simulink model "ship"  (Simulink 9.2)
settings: Solver=ode45  StartTime=0.0  StopTime=500  RelTol=1e-3  EnableMultiTasking=on
values from neighbouring files (symbols this model uses):
  K_pd = 0.8362    [variables.mat]
  psi_r = 30    [variables.mat]
  T_d = 72.5216    [variables.mat]
  T_f = 8.39    [variables.mat]
libraries: simulink x2, simulink_extras x2
settings Model: Creator=markh  LastModifiedBy=Kjetk
settings DataIOCC: SignalLoggingName=sigsOut
settings OptimizationCC: InitFltsAndDblsToZero=on
settings DebuggingCC: SaveWithParameterizedLinksMsg=none  SignalResolutionControl=TryResolveAllWithWarning  MultiTaskDSMMsg=warning  MultiTaskCondExecSysMsg=none
settings HardwareCC: TargetUnknown=on
settings GRTTargetCC: TargetFcnLib=ansi_tfl_tmw.mat

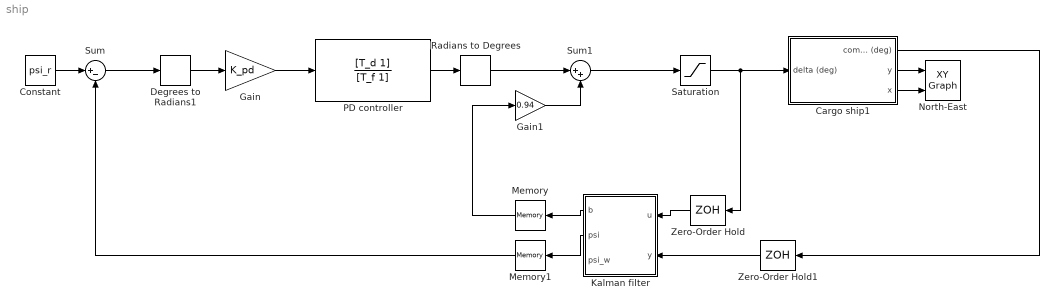
== system ship ==
  Cargo ship1 : Subsystem  mask(Simple shipmodel for a cargo ship){noise=on, current=on, logic=off}
      mask prompts: noise "measurement noise"; logic "waves"
      mask help:
      | Measurement noise:
      | 	checked = noise on
      | 	unchecked = noise off
      |
      | Current:
      | 	checked = current on
      | 	unchecked = current off
      |
      | Waves:
      | 	checked = waves on
      | 	unchecked = waves off
      |
      | Author: Jørgen Spjøtvold, 9/10-2003
      | TTK 4115 Linear system theory.
      | Modified by Jostein Bakkeheim 26/10-2006
  Constant : Constant  Value=psi_r
  Degrees to Radians1 : simulink_extras/Transformations/Degrees to Radians
  Gain : Gain  Gain=K_pd
  Gain1 : Gain  Gain=0.94
  Kalman filter : MATLAB Function  TreatAsAtomicUnit=on
  Memory : Memory
  Memory1 : Memory
  "North-East " : simulink/Sinks/XY Graph  xmin=-1  xmax=1  ymin=-1  ymax=1  st=-1
  PD controller : TransferFcn  Numerator=[T_d 1]  Denominator=[T_f 1]
  Radians to Degrees : simulink_extras/Transformations/Radians to Degrees
  Saturation : Saturate  UpperLimit=35  LowerLimit=-35
  Sum : Sum  Inputs=|+-
  Sum1 : Sum  Inputs=|++
  Zero-Order Hold : ZeroOrderHold  SampleTime=0.10
  Zero-Order Hold1 : ZeroOrderHold  SampleTime=0.10
  wires:
  Saturation/1 -> Cargo ship1/1(delta (deg)), Zero-Order Hold/1
  Degrees to Radians1/1 -> Gain/1
  Constant/1 -> Sum/1
  Sum/1 -> Degrees to Radians1/1
  Gain/1 -> PD controller/1
  PD controller/1 -> Radians to Degrees/1
  Cargo ship1/1(compass (deg)) -> Zero-Order Hold1/1
  Kalman filter/1(b) -> Memory/1
  Kalman filter/2(psi) -> Memory1/1
  Memory1/1 -> Sum/2
  Zero-Order Hold/1 -> Kalman filter/1(u)
  Zero-Order Hold1/1 -> Kalman filter/2(y)
  Memory/1 -> Gain1/1
  Sum1/1 -> Saturation/1
  Radians to Degrees/1 -> Sum1/1
  Gain1/1 -> Sum1/2
  Cargo ship1/2(y) -> "North-East "/1
  Cargo ship1/3(x) -> "North-East "/2

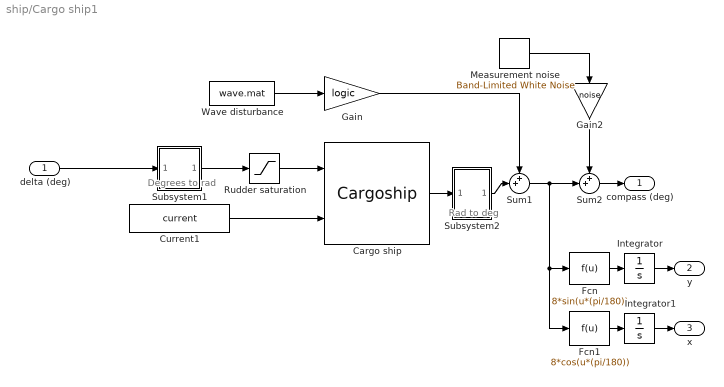
== system ship/Cargo ship1 ==
  note: Degrees to rad
  note: Rad to deg
  delta (deg) : Inport
  Cargo ship : S-Function  FunctionName=Cargoship  SFunctionDeploymentMode=off  EnableBusSupport=off  mask(Cargo ship){}
      mask help:
      | S-function which simulates a cargo ship.
      |
      | Author: Jørgen Spjøtvold
      | 20.10-2003
      | Modified by Jostein Bakkeheim 27.10.2006
  Current1 : Constant  Value=current
  Fcn : Fcn  Expr=8*sin(u*(pi/180))
  Fcn1 : Fcn  Expr=8*cos(u*(pi/180))
  Gain : Gain  Gain=logic  SaturateOnIntegerOverflow=on  OutDataTypeStr=Inherit: Same as input  ParamDataTypeStr=Inherit: Same as input
  Gain2 : Gain  Gain=noise  SaturateOnIntegerOverflow=on  OutDataTypeStr=Inherit: Same as input  ParamDataTypeStr=Inherit: Same as input
  Integrator : Integrator
  Integrator1 : Integrator
  Measurement noise : simulink/Sources/Band-Limited White Noise  Cov=[0.001]  Ts=.5  seed=[23341]
  Rudder saturation : Saturate  UpperLimit=45*(pi/180)  LowerLimit=-45*(pi/180)
  Subsystem1 : Subsystem  mask(degrees to radians){}
      mask help: Converts degrees to radians
      mask Display: fprintf('D2R');
  Subsystem2 : Subsystem  mask(radians to degrees){}
      mask help: Converts radians to degrees
      mask Display: fprintf('R2D');
  Sum1 : Sum  Inputs=++|  SaturateOnIntegerOverflow=on
  Sum2 : Sum  Inputs=++|  SaturateOnIntegerOverflow=on
  Wave disturbance : FromFile  FileName=wave.mat  SampleTime=0
  compass (deg) : Outport
  y : Outport  Port=2
  x : Outport  Port=3
  wires:
  delta (deg)/1 -> Subsystem1/1(In1)
  Fcn/1 -> Integrator/1
  Integrator/1 -> y/1
  Fcn1/1 -> Integrator1/1
  Integrator1/1 -> x/1
  Wave disturbance/1 -> Gain/1
  Subsystem2/1(Out1) -> Sum1/2
  Gain/1 -> Sum1/1
  Sum1/1 -> Fcn/1, Fcn1/1, Sum2/2
  Cargo ship/1 -> Subsystem2/1(In1)
  Subsystem1/1(Out1) -> Rudder saturation/1
  Rudder saturation/1 -> Cargo ship/1
  Sum2/1 -> compass (deg)/1
  Measurement noise/1 -> Gain2/1
  Gain2/1 -> Sum2/1
  Current1/1 -> Cargo ship/2

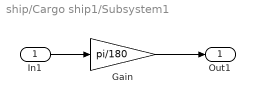
== system ship/Cargo ship1/Subsystem1 ==
  In1 : Inport
  Gain : Gain  Gain=pi/180  SaturateOnIntegerOverflow=on  OutDataTypeStr=Inherit: Same as input  ParamDataTypeStr=Inherit: Same as input
  Out1 : Outport
  wires:
  Gain/1 -> Out1/1
  In1/1 -> Gain/1

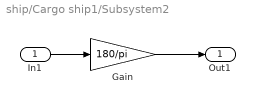
== system ship/Cargo ship1/Subsystem2 ==
  In1 : Inport
  Gain : Gain  Gain=180/pi  SaturateOnIntegerOverflow=on  OutDataTypeStr=Inherit: Same as input  ParamDataTypeStr=Inherit: Same as input
  Out1 : Outport
  wires:
  Gain/1 -> Out1/1
  In1/1 -> Gain/1

== matlab function Kalman filter ==
  data: u input double; b output double; y input double; psi output double; psi_w output double
function [b, psi, psi_w]= fcn(u,y)
persistent init_flag A_d B_d C_d E_d Q P_ x_ R

if isempty(init_flag)
    init_flag = 1;
    
    A_d = [0.997 0.0992 0 0 0;
           -0.0607 0.9830 0 0 0;
           0 0 1 0.0999 0;
           0 0 0 0.9986 -0.0002;
           0 0 0 0 1;
           ];
    B_d = 1.0e-03*[ 0
            0
            0.0108
            0.2151
            0
            ];
    C_d = [0 1 1 0 0];
    
        
    E_d = [0 0; 0.0004 0;
           0 0; 0 0; 0 0.1];
    
    Q = diag([30 10^(-7)]);

    P_ = diag([1 0.013 pi^2 1 0.0025]);
    
    x_ = [0; 0; 0; 0; 0];
    
    R = 6.1614 * 10^(-7)*10;
end



%compute kalman gain
L = P_*C_d'*(C_d*P_*C_d' + R)^(-1);

%update the estimate with the measurement
x = x_ + L*(y - C_d*x_);

%compute error covariance for updated estimator
I = diag([1 1 1 1 1 ]);
P = (I - L*C_d)*P_*(I-L*C_d)' + L*R*L';

%project ahead
P_ = A_d*P*A_d' + E_d*Q*E_d';
x_ = A_d*x + B_d*u;

psi = x(3);
b = x(5);
psi_w = x(2);
end
